simulink model "power_FCHPS_MEA"  (R2020b)
settings: Solver=ode23tb  StartTime=0.0  StopTime=350  RelTol=1e-3  EnableMultiTasking=on
PreLoadFcn:
  | Ts=100e-6;
InitFcn:
  | Ts=100e-6;
undefined symbols (not defined in the file or in its folder): DiscIntNeverNeededParam, Ion, Lithium
libraries: powerlib x93, simulink x8, powerlib_meascontrol x3, electricdrivelib x3
(part 2 of 4)

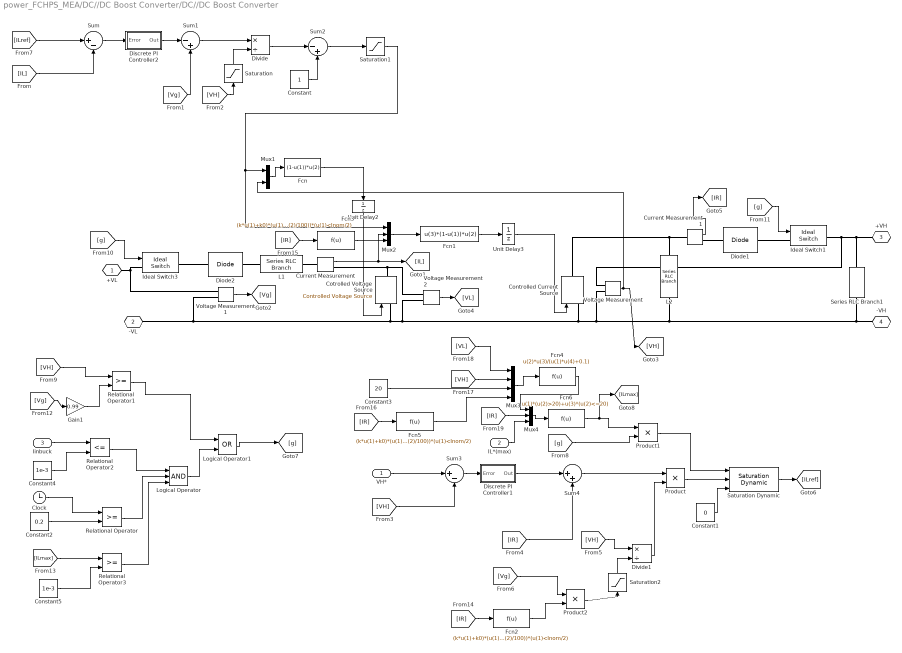
== system power_FCHPS_MEA/DC//DC Boost Converter/DC//DC Boost Converter ==
  VH* : Inport
  IL*(max) : Inport  Port=2
  Iinbuck : Inport  Port=3
  Clock : Clock
  Constant : Constant
  Constant1 : Constant  Value=0
  Constant2 : Constant  Value=0.2
  Constant3 : Constant  Value=20
  Constant4 : Constant  Value=1e-3
  Constant5 : Constant  Value=1e-3
  Controlled Current Source : powerlib/Electrical Sources/Controlled Current Source  Initialize=on  Source_Type=DC  Amplitude=0  Phase=0  Frequency=0  Measurements=None
  Cotrolled Voltage Source : powerlib/Electrical Sources/Controlled Voltage Source  Initialize=on  Source_Type=DC  Amplitude=0  Phase=0  Frequency=0  Measurements=None
  Current Measurement : powerlib/Measurements/Current Measurement  PhasorSimulation=off  OutputType=Complex  PSBequivalent=0
  Current Measurement1 : powerlib/Measurements/Current Measurement  PhasorSimulation=off  OutputType=Complex  PSBequivalent=0
  Diode1 : powerlib/Power Electronics/Diode  Ron=0.001  Lon=0  Vf=0  IC=0  UseSnubber=off  Rs=1e6  Cs=250e-9  Measurements=off
  Diode2 : powerlib/Power Electronics/Diode  Ron=0.001  Lon=0  Vf=0  IC=0  UseSnubber=off  Rs=1e6  Cs=250e-9  Measurements=off
  Discrete PI Controller1 : Subsystem  DialogController=POWERSYS.PowerSysDialog  mask(Discrete PI Controller){Kp=Kpv, Ki=Kiv, Par_Limits=[0.06 -0.06], Init=0, Ts=Ts}
      mask prompts: Kp "Proportional gain (Kp):"; Ki "Integral gain (Ki):"; Par_Limits "Output limits: [ Upper   Lower ]"; Init "Output initial value:"; Ts "Sample time:"
      mask help: This block implements a discrete PI controller.
      mask init:
      | UpperLimit=Par_Limits(1);
      | LowerLimit=Par_Limits(2);
      | power_initmask();
      mask Help: This block is part of a subset of blocks in the Extras library that does not have documentation associated with it, other than the block mask description.
      mask Display: disp('PI');
  Discrete PI Controller2 : Subsystem  DialogController=POWERSYS.PowerSysDialog  mask(Discrete PI Controller){Kp=Kpi, Ki=Kii, Par_Limits=[50 -50], Init=0, Ts=Ts}
      mask prompts: Kp "Proportional gain (Kp):"; Ki "Integral gain (Ki):"; Par_Limits "Output limits: [ Upper   Lower ]"; Init "Output initial value:"; Ts "Sample time:"
      mask help: This block implements a discrete PI controller.
      mask init:
      | UpperLimit=Par_Limits(1);
      | LowerLimit=Par_Limits(2);
      | power_initmask();
      mask Help: This block is part of a subset of blocks in the Extras library that does not have documentation associated with it, other than the block mask description.
      mask Display: disp('PI');
  Divide : Product  Inputs=*/  SampleTime=Ts
  Divide1 : Product  Inputs=*/  SampleTime=Ts
  Fcn : Fcn  Expr=(1-u(1))*u(2)
  Fcn1 : Fcn  Expr=u(3)*(1-u(1))*u(2)
  Fcn2 : Fcn  Expr=(k*u(1)+k0)*(u(1)>=Inom/2)+((n(2)/100))*(u(1)<Inom/2)  SampleTime=Ts
  Fcn3 : Fcn  Expr=(k*u(1)+k0)*(u(1)>=Inom/2)+((n(2)/100))*(u(1)<Inom/2)  SampleTime=Ts
  Fcn4 : Fcn  Expr=u(2)*u(3)/(u(1)*u(4)+0.1)  SampleTime=Ts
  Fcn5 : Fcn  Expr=(k*u(1)+k0)*(u(1)>=Inom/2)+((n(2)/100))*(u(1)<Inom/2)  SampleTime=Ts
  Fcn6 : Fcn  Expr=u(1)*(u(2)>20)+u(3)*(u(2)<=20)  SampleTime=Ts
  Gain1 : Gain  Gain=0.99  SampleTime=Ts
  Ideal Switch1 : powerlib/Power Electronics/Ideal Switch  Ron=0.001  Lon=0  IC=0  Rs=1e5  Cs=inf  Measurements=off
  Ideal Switch3 : powerlib/Power Electronics/Ideal Switch  Ron=0.001  Lon=0  IC=0  Rs=1e5  Cs=inf  Measurements=off
  L1 : powerlib/Elements/Series RLC Branch  LConnTagsString=__new0  RConnTagsString=__new0  BranchType=L  Resistance=0.3  Inductance=L  SetiL0=off  InitialCurrent=100  Capacitance=100e-6  Setx0=off  InitialVoltage=0  Measurements=None
  L2 : powerlib/Elements/Series RLC Branch  LConnTagsString=__new0  RConnTagsString=__new0  BranchType=RC  Resistance=0.01  Inductance=100e-6  SetiL0=off  InitialCurrent=100  Capacitance=800e-6  Setx0=off  InitialVoltage=0  Measurements=None
  Logical Operator : Logic  Inputs=3  AllPortsSameDT=off  OutDataTypeStr=boolean
  Logical Operator1 : Logic  Operator=OR  AllPortsSameDT=off  OutDataTypeStr=boolean
  Mux1 : Mux  Inputs=2
  Mux2 : Mux  Inputs=3
  Mux3 : Mux
  Mux4 : Mux  Inputs=3
  Product : Product  RndMeth=Zero
  Product1 : Product  RndMeth=Zero
  Product2 : Product  RndMeth=Zero
  Relational Operator : RelationalOperator  OutDataTypeStr=boolean  RndMeth=Nearest
  Relational Operator1 : RelationalOperator  OutDataTypeStr=boolean  RndMeth=Nearest
  Relational Operator2 : RelationalOperator  Operator=<=  OutDataTypeStr=boolean  RndMeth=Nearest
  Relational Operator3 : RelationalOperator  OutDataTypeStr=boolean  RndMeth=Nearest
  Saturation : Saturate  UpperLimit=inf  LowerLimit=0.01  SampleTime=Ts
  Saturation Dynamic : simulink/Discontinuities/Saturation Dynamic  OutMin=[]  OutMax=[]  OutDataTypeStr=Inherit: Same as second input  OutDataType=fixdt(1, 16)  OutScaling=2^-10  DoSatur=off
  Saturation1 : Saturate  UpperLimit=1  LowerLimit=0  SampleTime=Ts
  Saturation2 : Saturate  UpperLimit=inf  LowerLimit=0.01  SampleTime=Ts
  Series RLC Branch1 : powerlib/Elements/Series RLC Branch  LConnTagsString=__new0  RConnTagsString=__new0  BranchType=R  Resistance=5e3  Inductance=1e-3  SetiL0=off  InitialCurrent=0  Capacitance=15  Setx0=on  InitialVoltage=270  Measurements=None
  Sum : Sum  Inputs=|+-
  Sum1 : Sum  Inputs=|-+
  Sum2 : Sum  Inputs=|-+
  Sum3 : Sum  Inputs=|+-
  Sum4 : Sum  Inputs=|++
  Unit Delay2 : UnitDelay  SampleTime=Ts  HasFrameUpgradeWarning=on
  Unit Delay3 : UnitDelay  SampleTime=Ts  HasFrameUpgradeWarning=on
  Voltage Measurement : powerlib/Measurements/Voltage Measurement  PhasorSimulation=off  OutputType=Complex  PSBequivalent=0
  Voltage Measurement1 : powerlib/Measurements/Voltage Measurement  PhasorSimulation=off  OutputType=Complex  PSBequivalent=0
  Voltage Measurement2 : powerlib/Measurements/Voltage Measurement  PhasorSimulation=off  OutputType=Complex  PSBequivalent=0
  +VL : PMIOPort  Tag=PMCPort  Side=Left
  -VL : PMIOPort  Tag=PMCPort  Port=2  Side=Left
  +VH : PMIOPort  Tag=PMCPort  Port=3  Side=Right
  -VH : PMIOPort  Tag=PMCPort  Port=4  Side=Right
  wires:
  Voltage Measurement/1 -> [VH], Mux1/2
  Mux1/1 -> Fcn/1
  Fcn/1 -> Unit Delay2/1
  Current Measurement/1 -> Mux2/2, [IL]
  Mux2/1 -> Fcn1/1
  Voltage Measurement1/1 -> [Vg]
  [IL] -> Sum/2
  Sum/1 -> Discrete PI Controller2/1(Error)
  Discrete PI Controller2/1(Out) -> Sum1/1
  [Vg] -> Sum1/2
  Sum1/1 -> Divide/1
  [VH] -> Saturation/1
  Saturation/1 -> Divide/2
  Constant/1 -> Sum2/2
  Sum2/1 -> Saturation1/1
  Saturation1/1 -> Mux1/1, Mux2/1
  [VH] -> Sum3/2
  VH*/1 -> Sum3/1
  Sum3/1 -> Discrete PI Controller1/1(Error)
  Discrete PI Controller1/1(Out) -> Sum4/1
  [IR] -> Sum4/2
  Saturation2/1 -> Divide1/2
  Voltage Measurement2/1 -> [VL]
  Current Measurement1/1 -> [IR]
  Sum4/1 -> Product/1
  [VH] -> Divide1/1
  [Vg] -> Product2/1
  Product2/1 -> Saturation2/1
  Divide1/1 -> Product/2
  Product/1 -> Saturation Dynamic/2
  Constant1/1 -> Saturation Dynamic/3
  Saturation Dynamic/1 -> [ILref]
  Fcn1/1 -> Unit Delay3/1
  [g] -> Ideal Switch3/1
  [g] -> Ideal Switch1/1
  Clock/1 -> Relational Operator/1
  Constant2/1 -> Relational Operator/2
  [g] -> Product1/2
  [VH] -> Relational Operator1/1
  [Vg] -> Gain1/1
  Relational Operator1/1 -> Logical Operator1/1
  Gain1/1 -> Relational Operator1/2
  Product1/1 -> Saturation Dynamic/1
  Iinbuck/1 -> Relational Operator2/1
  Constant4/1 -> Relational Operator2/2
  Relational Operator2/1 -> Logical Operator/1
  Relational Operator/1 -> Logical Operator/2
  Logical Operator/1 -> Logical Operator1/2
  Logical Operator1/1 -> [g]
  [ILmax] -> Relational Operator3/1
  Constant5/1 -> Relational Operator3/2
  Relational Operator3/1 -> Logical Operator/3
  [ILref] -> Sum/1
  Fcn2/1 -> Product2/2
  [IR] -> Fcn3/1
  Fcn3/1 -> Mux2/3
  [IR] -> Fcn2/1
  Constant3/1 -> Mux3/3
  [VH] -> Mux3/2
  [VL] -> Mux3/1
  Mux3/1 -> Fcn4/1
  Fcn5/1 -> Mux3/4
  [IR] -> Fcn5/1
  Fcn4/1 -> Mux4/1
  [IR] -> Mux4/2
  IL*(max)/1 -> Mux4/3
  Mux4/1 -> Fcn6/1
  Fcn6/1 -> Product1/1, [ILmax]
  Unit Delay2/1 -> Cotrolled Voltage Source/1
  Unit Delay3/1 -> Controlled Current Source/1
  Divide/1 -> Sum2/1
  connections:
  Controlled Current Source/RConn1 -- L2/LConn1 -- Current Measurement1/LConn1
  Cotrolled Voltage Source/RConn1 -- Current Measurement/RConn1 -- Voltage Measurement2/LConn1
  L1/LConn1 -- Current Measurement/LConn1
  Diode2/RConn1 -- L1/RConn1
  Current Measurement1/RConn1 -- Diode1/LConn1
  -VH/RConn1 -- Controlled Current Source/LConn1 -- Voltage Measurement2/LConn2 -- Cotrolled Voltage Source/LConn1 -- Voltage Measurement1/LConn2 -- -VL/RConn1 -- Voltage Measurement/LConn2 -- L2/RConn1 -- Series RLC Branch1/RConn1
  Ideal Switch3/RConn1 -- Diode2/LConn1
  +VL/RConn1 -- Voltage Measurement1/LConn1 -- Ideal Switch3/LConn1
  Diode1/RConn1 -- Ideal Switch1/LConn1
  Voltage Measurement/LConn1 -- Ideal Switch1/RConn1 -- +VH/RConn1 -- Series RLC Branch1/LConn1

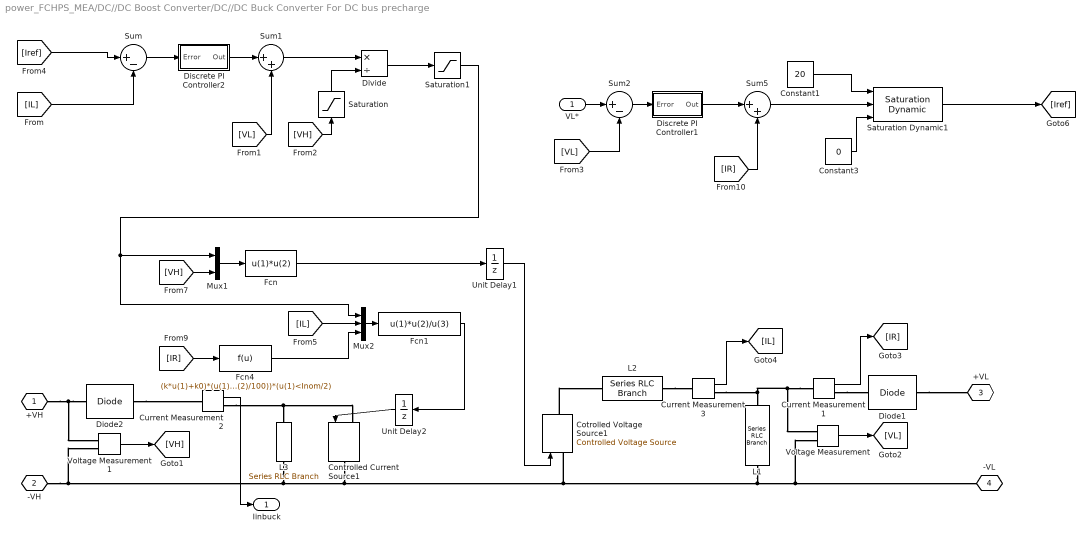
== system power_FCHPS_MEA/DC//DC Boost Converter/DC//DC Buck Converter For DC bus precharge ==
  VL* : Inport
  Constant1 : Constant  Value=20
  Constant3 : Constant  Value=0
  Controlled Current Source1 : powerlib/Electrical Sources/Controlled Current Source  Initialize=on  Source_Type=DC  Amplitude=0  Phase=0  Frequency=0  Measurements=None
  Cotrolled Voltage Source1 : powerlib/Electrical Sources/Controlled Voltage Source  Initialize=on  Source_Type=DC  Amplitude=0  Phase=0  Frequency=0  Measurements=None
  Current Measurement1 : powerlib/Measurements/Current Measurement  PhasorSimulation=off  OutputType=Complex  PSBequivalent=0
  Current Measurement2 : powerlib/Measurements/Current Measurement  PhasorSimulation=off  OutputType=Complex  PSBequivalent=0
  Current Measurement3 : powerlib/Measurements/Current Measurement  PhasorSimulation=off  OutputType=Complex  PSBequivalent=0
  Diode1 : powerlib/Power Electronics/Diode  Ron=0.001  Lon=0  Vf=0  IC=0  UseSnubber=off  Rs=1e6  Cs=250e-9  Measurements=off
  Diode2 : powerlib/Power Electronics/Diode  Ron=0.001  Lon=0  Vf=0  IC=0  UseSnubber=off  Rs=1e6  Cs=250e-9  Measurements=off
  Discrete PI Controller1 : Subsystem  DialogController=POWERSYS.PowerSysDialog  mask(Discrete PI Controller){Kp=Kpv, Ki=Kiv, Par_Limits=[1e6 -1e6], Init=0, Ts=Ts}
      mask prompts: Kp "Proportional gain (Kp):"; Ki "Integral gain (Ki):"; Par_Limits "Output limits: [ Upper   Lower ]"; Init "Output initial value:"; Ts "Sample time:"
      mask help: This block implements a discrete PI controller.
      mask init:
      | UpperLimit=Par_Limits(1);
      | LowerLimit=Par_Limits(2);
      | power_initmask();
      mask Help: This block is part of a subset of blocks in the Extras library that does not have documentation associated with it, other than the block mask description.
      mask Display: disp('PI');
  Discrete PI Controller2 : Subsystem  DialogController=POWERSYS.PowerSysDialog  mask(Discrete PI Controller){Kp=Kpi, Ki=Kii, Par_Limits=[1e6 -1e6], Init=0, Ts=Ts}
      mask prompts: Kp "Proportional gain (Kp):"; Ki "Integral gain (Ki):"; Par_Limits "Output limits: [ Upper   Lower ]"; Init "Output initial value:"; Ts "Sample time:"
      mask help: This block implements a discrete PI controller.
      mask init:
      | UpperLimit=Par_Limits(1);
      | LowerLimit=Par_Limits(2);
      | power_initmask();
      mask Help: This block is part of a subset of blocks in the Extras library that does not have documentation associated with it, other than the block mask description.
      mask Display: disp('PI');
  Divide : Product  Inputs=*/  SampleTime=Ts
  Fcn : Fcn  Expr=u(1)*u(2)
  Fcn1 : Fcn  Expr=u(1)*u(2)/u(3)
  Fcn4 : Fcn  Expr=(k*u(1)+k0)*(u(1)>=Inom/2)+((n(2)/100))*(u(1)<Inom/2)  SampleTime=Ts
  L1 : powerlib/Elements/Series RLC Branch  LConnTagsString=__new0  RConnTagsString=__new0  BranchType=RC  Resistance=0.01  Inductance=10e-6  SetiL0=off  InitialCurrent=100  Capacitance=800e-6  Setx0=off  InitialVoltage=0  Measurements=None
  L2 : powerlib/Elements/Series RLC Branch  LConnTagsString=__new0  RConnTagsString=__new0  BranchType=L  Resistance=0.3  Inductance=L  SetiL0=off  InitialCurrent=100  Capacitance=100e-6  Setx0=off  InitialVoltage=0  Measurements=None
  L3 : powerlib/Elements/Series RLC Branch  LConnTagsString=__new0  RConnTagsString=__new0  BranchType=R  Resistance=1e6  Inductance=10e-6  SetiL0=off  InitialCurrent=100  Capacitance=800e-6  Setx0=off  InitialVoltage=0  Measurements=None
  Mux1 : Mux  Inputs=2
  Mux2 : Mux  Inputs=3
  Saturation : Saturate  UpperLimit=inf  LowerLimit=0.01  SampleTime=Ts
  Saturation Dynamic1 : simulink/Discontinuities/Saturation Dynamic  OutMin=[]  OutMax=[]  OutDataTypeStr=Inherit: Same as second input  OutDataType=fixdt(1, 16)  OutScaling=2^-10  DoSatur=off
  Saturation1 : Saturate  UpperLimit=1  LowerLimit=0  SampleTime=Ts
  Sum : Sum  Inputs=|+-
  Sum1 : Sum  Inputs=|++
  Sum2 : Sum  Inputs=|+-
  Sum5 : Sum  Inputs=|++
  Unit Delay1 : UnitDelay  SampleTime=Ts  HasFrameUpgradeWarning=on
  Unit Delay2 : UnitDelay  SampleTime=Ts  HasFrameUpgradeWarning=on
  Voltage Measurement : powerlib/Measurements/Voltage Measurement  PhasorSimulation=off  OutputType=Complex  PSBequivalent=0
  Voltage Measurement1 : powerlib/Measurements/Voltage Measurement  PhasorSimulation=off  OutputType=Complex  PSBequivalent=0
  +VH : PMIOPort  Tag=PMCPort  Side=Left
  -VH : PMIOPort  Tag=PMCPort  Port=2  Side=Left
  +VL : PMIOPort  Tag=PMCPort  Port=3  Side=Right
  -VL : PMIOPort  Tag=PMCPort  Port=4  Side=Right
  Iinbuck : Outport  VectorParamsAs1DForOutWhenUnconnected=off
  wires:
  Mux2/1 -> Fcn1/1
  Mux1/1 -> Fcn/1
  Voltage Measurement/1 -> [VL]
  Voltage Measurement1/1 -> [VH]
  Current Measurement2/1 -> Iinbuck/1
  Current Measurement1/1 -> [IR]
  [IL] -> Mux2/2
  [VH] -> Mux1/2
  Fcn/1 -> Unit Delay1/1
  Fcn1/1 -> Unit Delay2/1
  [IL] -> Sum/2
  Sum/1 -> Discrete PI Controller2/1(Error)
  Discrete PI Controller2/1(Out) -> Sum1/1
  [VL] -> Sum1/2
  Sum1/1 -> Divide/1
  [VH] -> Saturation/1
  Saturation/1 -> Divide/2
  Divide/1 -> Saturation1/1
  Saturation1/1 -> Mux2/1, Mux1/1
  [Iref] -> Sum/1
  Sum2/1 -> Discrete PI Controller1/1(Error)
  Discrete PI Controller1/1(Out) -> Sum5/1
  [IR] -> Sum5/2
  Sum5/1 -> Saturation Dynamic1/2
  Constant3/1 -> Saturation Dynamic1/3
  Saturation Dynamic1/1 -> [Iref]
  VL*/1 -> Sum2/1
  [VL] -> Sum2/2
  Current Measurement3/1 -> [IL]
  [IR] -> Fcn4/1
  Fcn4/1 -> Mux2/3
  Constant1/1 -> Saturation Dynamic1/1
  Unit Delay1/1 -> Cotrolled Voltage Source1/1
  Unit Delay2/1 -> Controlled Current Source1/1
  connections:
  -VH/RConn1 -- Voltage Measurement1/LConn2 -- Cotrolled Voltage Source1/LConn1 -- L1/RConn1 -- -VL/RConn1 -- Voltage Measurement/LConn2 -- Controlled Current Source1/RConn1 -- L3/RConn1
  Diode2/LConn1 -- +VH/RConn1 -- Voltage Measurement1/LConn1
  Cotrolled Voltage Source1/RConn1 -- L2/RConn1
  Current Measurement1/LConn1 -- Voltage Measurement/LConn1 -- Current Measurement3/RConn1 -- L1/LConn1
  Current Measurement1/RConn1 -- Diode1/LConn1
  Diode1/RConn1 -- +VL/RConn1
  Current Measurement2/RConn1 -- Controlled Current Source1/LConn1 -- L3/LConn1
  L2/LConn1 -- Current Measurement3/LConn1
  Diode2/RConn1 -- Current Measurement2/LConn1

== system power_FCHPS_MEA/DC//DC Buck Converter/Discrete PI Controller1 ==
  note: Discrete PID Controller
  note: Pierre Giroux, Gilbert Sybille
      | Power System Simulation Laboratory
      | IREQ, Hydro-Quebc
  Error : Inport  SampleTime=Ts
  Discrete-Time Integrator : DiscreteIntegrator  InitialCondition=Init  SampleTime=Ts  LimitOutput=on  UpperSaturationLimit=UpperLimit  LowerSaturationLimit=LowerLimit  ICPrevOutput=DiscIntNeverNeededParam  ICPrevScaledInput=DiscIntNeverNeededParam
  Kp4 : Gain  Gain=Kp  SaturateOnIntegerOverflow=on  SampleTime=Ts  OutDataTypeStr=Inherit: Same as input  ParamDataTypeStr=Inherit: Same as input
  Kp5 : Gain  Gain=Ki  SaturateOnIntegerOverflow=on  SampleTime=Ts  OutDataTypeStr=Inherit: Same as input  ParamDataTypeStr=Inherit: Same as input
  Saturation2 : Saturate  UpperLimit=UpperLimit  LowerLimit=LowerLimit  SampleTime=Ts
  Sum6 : Sum  InputSameDT=on  SaturateOnIntegerOverflow=on  SampleTime=Ts  OutDataTypeStr=Inherit: Same as first input
  Zero-Order Hold : ZeroOrderHold  SampleTime=Ts
  Out : Outport  SampleTime=Ts  InitialOutput=0  VectorParamsAs1DForOutWhenUnconnected=off
  wires:
  Zero-Order Hold/1 -> Sum6/1
  Saturation2/1 -> Out/1
  Discrete-Time Integrator/1 -> Sum6/2
  Kp4/1 -> Zero-Order Hold/1
  Kp5/1 -> Discrete-Time Integrator/1
  Sum6/1 -> Saturation2/1
  Error/1 -> Kp5/1, Kp4/1

== system power_FCHPS_MEA/DC//DC Buck Converter/Discrete PI Controller2 ==
  note: Pierre Giroux, Gilbert Sybille
      | Power System Simulation Laboratory
      | IREQ, Hydro-Quebc
  note: Discrete PID Controller
  Error : Inport  SampleTime=Ts
  Discrete-Time Integrator : DiscreteIntegrator  InitialCondition=Init  SampleTime=Ts  LimitOutput=on  UpperSaturationLimit=UpperLimit  LowerSaturationLimit=LowerLimit  ICPrevOutput=DiscIntNeverNeededParam  ICPrevScaledInput=DiscIntNeverNeededParam
  Kp4 : Gain  Gain=Kp  SaturateOnIntegerOverflow=on  SampleTime=Ts  OutDataTypeStr=Inherit: Same as input  ParamDataTypeStr=Inherit: Same as input
  Kp5 : Gain  Gain=Ki  SaturateOnIntegerOverflow=on  SampleTime=Ts  OutDataTypeStr=Inherit: Same as input  ParamDataTypeStr=Inherit: Same as input
  Saturation2 : Saturate  UpperLimit=UpperLimit  LowerLimit=LowerLimit  SampleTime=Ts
  Sum6 : Sum  InputSameDT=on  SaturateOnIntegerOverflow=on  SampleTime=Ts  OutDataTypeStr=Inherit: Same as first input
  Zero-Order Hold : ZeroOrderHold  SampleTime=Ts
  Out : Outport  SampleTime=Ts  InitialOutput=0  VectorParamsAs1DForOutWhenUnconnected=off
  wires:
  Error/1 -> Kp4/1, Kp5/1
  Sum6/1 -> Saturation2/1
  Kp5/1 -> Discrete-Time Integrator/1
  Kp4/1 -> Zero-Order Hold/1
  Discrete-Time Integrator/1 -> Sum6/2
  Saturation2/1 -> Out/1
  Zero-Order Hold/1 -> Sum6/1

== system power_FCHPS_MEA/Energy Management System/Battery DC//DC charge converter reference ==
  IBAT* : Inport
  Constant1 : Constant  Value=0
  Constant8 : Constant  Value=58
  Switch5 : Switch  Criteria=u2 > Threshold
  IBAT_maxC* : Outport  VectorParamsAs1DForOutWhenUnconnected=off
  VBAT* : Outport  Port=2  VectorParamsAs1DForOutWhenUnconnected=off
  wires:
  [EMSON] -> Switch5/2
  IBAT*/1 -> Switch5/1
  Constant1/1 -> Switch5/3
  Switch5/1 -> IBAT_maxC*/1
  Constant8/1 -> VBAT*/1

== system power_FCHPS_MEA/Energy Management System/Battery DC//DC discharge converter references  ==
  IBAT* : Inport
  Constant10 : Constant  Value=0
  Constant6 : Constant  Value=270
  Switch1 : Switch  Criteria=u2 > Threshold
  Switch10 : Switch  Criteria=u2 > Threshold
  IBAT_maxD* : Outport  VectorParamsAs1DForOutWhenUnconnected=off
  VDC2* : Outport  Port=2  VectorParamsAs1DForOutWhenUnconnected=off
  wires:
  Switch10/1 -> VDC2*/1
  [EMSON] -> Switch10/2
  Constant6/1 -> Switch10/3
  IBAT*/1 -> Switch1/1
  [Vdcref] -> Switch10/1
  [EMSON] -> Switch1/2
  Switch1/1 -> IBAT_maxD*/1
  Constant10/1 -> Switch1/3

== system power_FCHPS_MEA/Energy Management System/FC DC//DC converter references ==
  IFC* : Inport
  Add1 : Sum  Inputs=+-
  Constant11 : Constant  Value=212
  Constant22 : Constant  Value=270
  Constant3 : Constant  Value=15
  Constant4 : Constant  Value=297
  Constant7 : Constant  Value=250
  Fcn : Fcn  Expr=u(1)*(u(1)<u(2))+u(2)*(u(1)>=u(2))
  Mux6 : Mux  Inputs=2
  Relational Operator6 : RelationalOperator  Operator=<=  OutDataTypeStr=boolean  RndMeth=Nearest
  Switch : Switch  Criteria=u2 > Threshold
  Switch6 : Switch  Criteria=u2 > Threshold
  Switch9 : Switch  Criteria=u2 > Threshold
  filter : Subsystem
  IFC*max : Outport  VectorParamsAs1DForOutWhenUnconnected=off
  VDC1* : Outport  Port=2  VectorParamsAs1DForOutWhenUnconnected=off
  wires:
  [EMSON] -> Switch9/2
  Switch9/1 -> VDC1*/1
  Constant4/1 -> Switch9/1
  Constant22/1 -> Switch9/3
  Switch6/1 -> Switch/1
  Constant11/1 -> Relational Operator6/2, Switch6/3
  Relational Operator6/1 -> Switch6/2
  Constant7/1 -> Switch/3
  Constant3/1 -> Add1/2
  IFC*/1 -> Relational Operator6/1, Switch6/1
  Mux6/1 -> Fcn/1
  Fcn/1 -> filter/1(I)
  [EMSON] -> Switch/2
  Switch/1 -> Mux6/1
  filter/1(If) -> IFC*max/1
  Add1/1 -> Mux6/2
  [IFCAllow] -> Add1/1

== system power_FCHPS_MEA/Energy Management System/Load Disconnect ==
  SOC : Inport
  Vdc : Inport  Port=2
  Constant17 : Constant  Value=40
  Constant18 : Constant  Value=0
  Constant19 : Constant  Value=0
  Constant2 : Constant  Value=270
  Constant5 : Constant
  Constant9 : Constant  Value=200
  Data Type Conversion2 : DataTypeConversion
  Logical Operator3 : Logic  AllPortsSameDT=off  OutDataTypeStr=boolean
  Relational Operator : RelationalOperator  OutDataTypeStr=boolean  RndMeth=Nearest
  Relational Operator3 : RelationalOperator  Operator=<=  OutDataTypeStr=boolean  RndMeth=Nearest
  Relational Operator5 : RelationalOperator  Operator=<=  OutDataTypeStr=boolean  RndMeth=Nearest
  Switch2 : Switch  Criteria=u2 > Threshold
  Switch7 : Switch  Criteria=u2 > Threshold
  Switch8 : Switch  Criteria=u2 > Threshold
  Unit Delay : UnitDelay  SampleTime=Ts  HasFrameUpgradeWarning=on
  Unit Delay4 : UnitDelay  InitialCondition=1  SampleTime=Ts  HasFrameUpgradeWarning=on
  LoadON : Outport  VectorParamsAs1DForOutWhenUnconnected=off
  tag scope: EMSON=global
  wires:
  Data Type Conversion2/1 -> LoadON/1
  Relational Operator3/1 -> Switch8/2
  Constant18/1 -> Switch7/1
  Switch8/1 -> Switch2/3
  Relational Operator5/1 -> Switch7/2
  Constant17/1 -> Relational Operator5/2
  Switch7/1 -> Unit Delay4/1, Logical Operator3/1
  Unit Delay4/1 -> Switch7/3
  Unit Delay/1 -> Switch8/3
  SOC/1 -> Relational Operator5/1
  Logical Operator3/1 -> Data Type Conversion2/1
  Constant19/1 -> Switch8/1
  Constant9/1 -> Relational Operator3/2
  Relational Operator/1 -> Switch2/2
  Constant5/1 -> Switch2/1
  Constant2/1 -> Relational Operator/2
  Switch2/1 -> [EMSON], Unit Delay/1, Logical Operator3/2
  Vdc/1 -> Relational Operator/1, Relational Operator3/1

== system power_FCHPS_MEA/Energy Management System/Model ==
  Pload : Inport
  SOC : Inport  Port=2
  Classical PI Control : Subsystem  VariantControl=ClassicalPI
  ECMS Control : Subsystem  VariantControl=ECMS
  EEMS Control : Subsystem  VariantControl=EEMS
  Frequency Decoupling and State Machine Control : Subsystem  VariantControl=FrequencyDecoupling
  State Machine Control : Subsystem  VariantControl=RuleBasedFuzzyLogic
  IFC* : Outport  VectorParamsAs1DForOutWhenUnconnected=off
  IBATD* : Outport  Port=2  VectorParamsAs1DForOutWhenUnconnected=off
  IBATC* : Outport  Port=3  VectorParamsAs1DForOutWhenUnconnected=off

== system power_FCHPS_MEA/Energy Management System/Protecting resistor connect ==
  Vdc : Inport
  Constant12 : Constant  Value=290
  Constant13 : Constant
  Constant14 : Constant  Value=285
  Constant15 : Constant  Value=0
  Data Type Conversion1 : DataTypeConversion
  Relational Operator1 : RelationalOperator  OutDataTypeStr=boolean  RndMeth=Nearest
  Relational Operator2 : RelationalOperator  Operator=<=  OutDataTypeStr=boolean  RndMeth=Nearest
  Switch3 : Switch  Criteria=u2 > Threshold
  Switch4 : Switch  Criteria=u2 > Threshold
  Unit Delay1 : UnitDelay  SampleTime=Ts  HasFrameUpgradeWarning=on
  ResON : Outport  VectorParamsAs1DForOutWhenUnconnected=off
  wires:
  Unit Delay1/1 -> Switch4/3
  Vdc/1 -> Relational Operator1/1, Relational Operator2/1
  Switch4/1 -> Switch3/3
  Switch3/1 -> Data Type Conversion1/1, Unit Delay1/1
  Relational Operator1/1 -> Switch3/2
  Relational Operator2/1 -> Switch4/2
  Data Type Conversion1/1 -> ResON/1
  Constant15/1 -> Switch4/1
  Constant13/1 -> Switch3/1
  Constant14/1 -> Relational Operator2/2
  Constant12/1 -> Relational Operator1/2

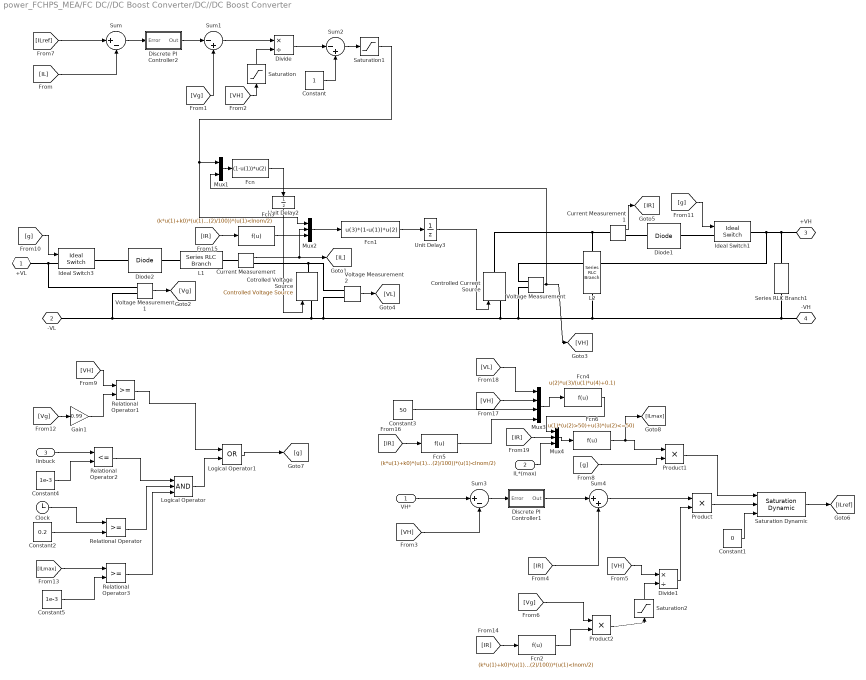
== system power_FCHPS_MEA/FC DC//DC Boost Converter/DC//DC Boost Converter ==
  VH* : Inport
  IL*(max) : Inport  Port=2
  Iinbuck : Inport  Port=3
  Clock : Clock
  Constant : Constant
  Constant1 : Constant  Value=0
  Constant2 : Constant  Value=0.2
  Constant3 : Constant  Value=50
  Constant4 : Constant  Value=1e-3
  Constant5 : Constant  Value=1e-3
  Controlled Current Source : powerlib/Electrical Sources/Controlled Current Source  Initialize=on  Source_Type=DC  Amplitude=0  Phase=0  Frequency=0  Measurements=None
  Cotrolled Voltage Source : powerlib/Electrical Sources/Controlled Voltage Source  Initialize=on  Source_Type=DC  Amplitude=0  Phase=0  Frequency=0  Measurements=None
  Current Measurement : powerlib/Measurements/Current Measurement  PhasorSimulation=off  OutputType=Complex  PSBequivalent=0
  Current Measurement1 : powerlib/Measurements/Current Measurement  PhasorSimulation=off  OutputType=Complex  PSBequivalent=0
  Diode1 : powerlib/Power Electronics/Diode  Ron=0.001  Lon=0  Vf=0  IC=0  UseSnubber=off  Rs=1e6  Cs=250e-9  Measurements=off
  Diode2 : powerlib/Power Electronics/Diode  Ron=0.001  Lon=0  Vf=0  IC=0  UseSnubber=off  Rs=1e6  Cs=250e-9  Measurements=off
  Discrete PI Controller1 : Subsystem  DialogController=POWERSYS.PowerSysDialog  mask(Discrete PI Controller){Kp=Kpv, Ki=Kiv, Par_Limits=[0.5 -0.5], Init=0, Ts=Ts}
      mask prompts: Kp "Proportional gain (Kp):"; Ki "Integral gain (Ki):"; Par_Limits "Output limits: [ Upper   Lower ]"; Init "Output initial value:"; Ts "Sample time:"
      mask help: This block implements a discrete PI controller.
      mask init:
      | UpperLimit=Par_Limits(1);
      | LowerLimit=Par_Limits(2);
      | power_initmask();
      mask Help: This block is part of a subset of blocks in the Extras library that does not have documentation associated with it, other than the block mask description.
      mask Display: disp('PI');
  Discrete PI Controller2 : Subsystem  DialogController=POWERSYS.PowerSysDialog  mask(Discrete PI Controller){Kp=Kpi/1000, Ki=Kii/1000, Par_Limits=[50 -50], Init=0, Ts=Ts}
      mask prompts: Kp "Proportional gain (Kp):"; Ki "Integral gain (Ki):"; Par_Limits "Output limits: [ Upper   Lower ]"; Init "Output initial value:"; Ts "Sample time:"
      mask help: This block implements a discrete PI controller.
      mask init:
      | UpperLimit=Par_Limits(1);
      | LowerLimit=Par_Limits(2);
      | power_initmask();
      mask Help: This block is part of a subset of blocks in the Extras library that does not have documentation associated with it, other than the block mask description.
      mask Display: disp('PI');
  Divide : Product  Inputs=*/  SampleTime=Ts
  Divide1 : Product  Inputs=*/  SampleTime=Ts
  Fcn : Fcn  Expr=(1-u(1))*u(2)
  Fcn1 : Fcn  Expr=u(3)*(1-u(1))*u(2)
  Fcn2 : Fcn  Expr=(k*u(1)+k0)*(u(1)>=Inom/2)+((n(2)/100))*(u(1)<Inom/2)  SampleTime=Ts
  Fcn3 : Fcn  Expr=(k*u(1)+k0)*(u(1)>=Inom/2)+((n(2)/100))*(u(1)<Inom/2)  SampleTime=Ts
  Fcn4 : Fcn  Expr=u(2)*u(3)/(u(1)*u(4)+0.1)  SampleTime=Ts
  Fcn5 : Fcn  Expr=(k*u(1)+k0)*(u(1)>=Inom/2)+((n(2)/100))*(u(1)<Inom/2)  SampleTime=Ts
  Fcn6 : Fcn  Expr=u(1)*(u(2)>50)+u(3)*(u(2)<=50)  SampleTime=Ts
  Gain1 : Gain  Gain=0.99  SampleTime=Ts
  Ideal Switch1 : powerlib/Power Electronics/Ideal Switch  Ron=0.001  Lon=0  IC=0  Rs=1e5  Cs=inf  Measurements=off
  Ideal Switch3 : powerlib/Power Electronics/Ideal Switch  Ron=0.001  Lon=0  IC=0  Rs=1e5  Cs=inf  Measurements=off
  L1 : powerlib/Elements/Series RLC Branch  LConnTagsString=__new0  RConnTagsString=__new0  BranchType=L  Resistance=0.3  Inductance=L  SetiL0=off  InitialCurrent=100  Capacitance=100e-6  Setx0=off  InitialVoltage=0  Measurements=None
  L2 : powerlib/Elements/Series RLC Branch  LConnTagsString=__new0  RConnTagsString=__new0  BranchType=RC  Resistance=0.01  Inductance=100e-6  SetiL0=off  InitialCurrent=100  Capacitance=800e-6  Setx0=off  InitialVoltage=0  Measurements=None
  Logical Operator : Logic  Inputs=3  AllPortsSameDT=off  OutDataTypeStr=boolean
  Logical Operator1 : Logic  Operator=OR  AllPortsSameDT=off  OutDataTypeStr=boolean
  Mux1 : Mux  Inputs=2
  Mux2 : Mux  Inputs=3
  Mux3 : Mux
  Mux4 : Mux  Inputs=3
  Product : Product  RndMeth=Zero
  Product1 : Product  RndMeth=Zero
  Product2 : Product  RndMeth=Zero
  Relational Operator : RelationalOperator  OutDataTypeStr=boolean  RndMeth=Nearest
  Relational Operator1 : RelationalOperator  OutDataTypeStr=boolean  RndMeth=Nearest
  Relational Operator2 : RelationalOperator  Operator=<=  OutDataTypeStr=boolean  RndMeth=Nearest
  Relational Operator3 : RelationalOperator  OutDataTypeStr=boolean  RndMeth=Nearest
  Saturation : Saturate  UpperLimit=inf  LowerLimit=0.01  SampleTime=Ts
  Saturation Dynamic : simulink/Discontinuities/Saturation Dynamic  OutMin=[]  OutMax=[]  OutDataTypeStr=Inherit: Same as second input  OutDataType=fixdt(1, 16)  OutScaling=2^-10  DoSatur=off
  Saturation1 : Saturate  UpperLimit=1  LowerLimit=0  SampleTime=Ts
  Saturation2 : Saturate  UpperLimit=inf  LowerLimit=0.01  SampleTime=Ts
  Series RLC Branch1 : powerlib/Elements/Series RLC Branch  LConnTagsString=__new0  RConnTagsString=__new0  BranchType=R  Resistance=5e3  Inductance=1e-3  SetiL0=off  InitialCurrent=0  Capacitance=15  Setx0=on  InitialVoltage=270  Measurements=None
  Sum : Sum  Inputs=|+-
  Sum1 : Sum  Inputs=|-+
  Sum2 : Sum  Inputs=|-+
  Sum3 : Sum  Inputs=|+-
  Sum4 : Sum  Inputs=|++
  Unit Delay2 : UnitDelay  SampleTime=Ts  HasFrameUpgradeWarning=on
  Unit Delay3 : UnitDelay  SampleTime=Ts  HasFrameUpgradeWarning=on
  Voltage Measurement : powerlib/Measurements/Voltage Measurement  PhasorSimulation=off  OutputType=Complex  PSBequivalent=0
  Voltage Measurement1 : powerlib/Measurements/Voltage Measurement  PhasorSimulation=off  OutputType=Complex  PSBequivalent=0
  Voltage Measurement2 : powerlib/Measurements/Voltage Measurement  PhasorSimulation=off  OutputType=Complex  PSBequivalent=0
  +VL : PMIOPort  Tag=PMCPort  Side=Left
  -VL : PMIOPort  Tag=PMCPort  Port=2  Side=Left
  +VH : PMIOPort  Tag=PMCPort  Port=3  Side=Right
  -VH : PMIOPort  Tag=PMCPort  Port=4  Side=Right
  wires:
  Unit Delay3/1 -> Controlled Current Source/1
  Unit Delay2/1 -> Cotrolled Voltage Source/1
  Fcn6/1 -> [ILmax], Product1/1
  Mux4/1 -> Fcn6/1
  IL*(max)/1 -> Mux4/3
  [IR] -> Mux4/2
  Fcn4/1 -> Mux4/1
  [IR] -> Fcn5/1
  Fcn5/1 -> Mux3/4
  Mux3/1 -> Fcn4/1
  [VL] -> Mux3/1
  [VH] -> Mux3/2
  Constant3/1 -> Mux3/3
  [IR] -> Fcn2/1
  Fcn3/1 -> Mux2/3
  Fcn2/1 -> Product2/2
  [ILref] -> Sum/1
  Relational Operator3/1 -> Logical Operator/3
  Constant5/1 -> Relational Operator3/2
  [ILmax] -> Relational Operator3/1
  Logical Operator1/1 -> [g]
  Logical Operator/1 -> Logical Operator1/2
  Relational Operator/1 -> Logical Operator/2
  Relational Operator2/1 -> Logical Operator/1
  Constant4/1 -> Relational Operator2/2
  Iinbuck/1 -> Relational Operator2/1
  Product1/1 -> Saturation Dynamic/1
  Gain1/1 -> Relational Operator1/2
  Relational Operator1/1 -> Logical Operator1/1
  [Vg] -> Gain1/1
  [VH] -> Relational Operator1/1
  [g] -> Product1/2
  Constant2/1 -> Relational Operator/2
  Clock/1 -> Relational Operator/1
  [g] -> Ideal Switch1/1
  [g] -> Ideal Switch3/1
  Fcn1/1 -> Unit Delay3/1
  Saturation Dynamic/1 -> [ILref]
  Constant1/1 -> Saturation Dynamic/3
  Product/1 -> Saturation Dynamic/2
  Divide1/1 -> Product/2
  Product2/1 -> Saturation2/1
  [Vg] -> Product2/1
  [VH] -> Divide1/1
  Sum4/1 -> Product/1
  Current Measurement1/1 -> [IR]
  Voltage Measurement2/1 -> [VL]
  Saturation2/1 -> Divide1/2
  [IR] -> Sum4/2
  Discrete PI Controller1/1(Out) -> Sum4/1
  Sum3/1 -> Discrete PI Controller1/1(Error)
  VH*/1 -> Sum3/1
  [VH] -> Sum3/2
  Sum2/1 -> Saturation1/1
  Constant/1 -> Sum2/2
  Saturation/1 -> Divide/2
  [VH] -> Saturation/1
  Sum1/1 -> Divide/1
  [Vg] -> Sum1/2
  Discrete PI Controller2/1(Out) -> Sum1/1
  Sum/1 -> Discrete PI Controller2/1(Error)
  [IL] -> Sum/2
  Voltage Measurement1/1 -> [Vg]
  Mux2/1 -> Fcn1/1
  Current Measurement/1 -> [IL], Mux2/2
  Fcn/1 -> Unit Delay2/1
  Mux1/1 -> Fcn/1
  Voltage Measurement/1 -> [VH], Mux1/2
  [IR] -> Fcn3/1
  Divide/1 -> Sum2/1
  Saturation1/1 -> Mux2/1, Mux1/1
  connections:
  Series RLC Branch1/LConn1 -- +VH/RConn1 -- Ideal Switch1/RConn1 -- Voltage Measurement/LConn1
  Diode1/RConn1 -- Ideal Switch1/LConn1
  +VL/RConn1 -- Voltage Measurement1/LConn1 -- Ideal Switch3/LConn1
  Ideal Switch3/RConn1 -- Diode2/LConn1
  Series RLC Branch1/RConn1 -- L2/RConn1 -- Voltage Measurement/LConn2 -- -VL/RConn1 -- Voltage Measurement1/LConn2 -- Cotrolled Voltage Source/LConn1 -- Voltage Measurement2/LConn2 -- Controlled Current Source/LConn1 -- -VH/RConn1
  Current Measurement1/RConn1 -- Diode1/LConn1
  Diode2/RConn1 -- L1/RConn1
  L1/LConn1 -- Current Measurement/LConn1
  Current Measurement/RConn1 -- Voltage Measurement2/LConn1 -- Cotrolled Voltage Source/RConn1
  Current Measurement1/LConn1 -- L2/LConn1 -- Controlled Current Source/RConn1

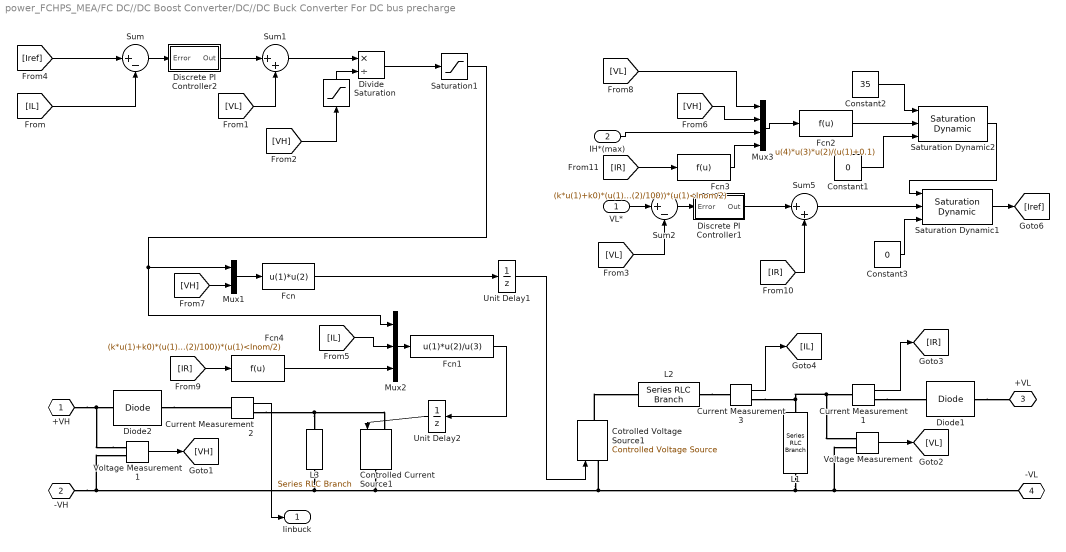
== system power_FCHPS_MEA/FC DC//DC Boost Converter/DC//DC Buck Converter For DC bus precharge ==
  VL* : Inport
  IH*(max) : Inport  Port=2
  Constant1 : Constant  Value=0
  Constant2 : Constant  Value=35
  Constant3 : Constant  Value=0
  Controlled Current Source1 : powerlib/Electrical Sources/Controlled Current Source  Initialize=on  Source_Type=DC  Amplitude=0  Phase=0  Frequency=0  Measurements=None
  Cotrolled Voltage Source1 : powerlib/Electrical Sources/Controlled Voltage Source  Initialize=on  Source_Type=DC  Amplitude=0  Phase=0  Frequency=0  Measurements=None
  Current Measurement1 : powerlib/Measurements/Current Measurement  PhasorSimulation=off  OutputType=Complex  PSBequivalent=0
  Current Measurement2 : powerlib/Measurements/Current Measurement  PhasorSimulation=off  OutputType=Complex  PSBequivalent=0
  Current Measurement3 : powerlib/Measurements/Current Measurement  PhasorSimulation=off  OutputType=Complex  PSBequivalent=0
  Diode1 : powerlib/Power Electronics/Diode  Ron=0.001  Lon=0  Vf=0  IC=0  UseSnubber=off  Rs=1e6  Cs=250e-9  Measurements=off
  Diode2 : powerlib/Power Electronics/Diode  Ron=0.001  Lon=0  Vf=0  IC=0  UseSnubber=off  Rs=1e6  Cs=250e-9  Measurements=off
  Discrete PI Controller1 : Subsystem  DialogController=POWERSYS.PowerSysDialog  mask(Discrete PI Controller){Kp=Kpv, Ki=Kiv, Par_Limits=[1e6 -1e6], Init=0, Ts=Ts}
      mask prompts: Kp "Proportional gain (Kp):"; Ki "Integral gain (Ki):"; Par_Limits "Output limits: [ Upper   Lower ]"; Init "Output initial value:"; Ts "Sample time:"
      mask help: This block implements a discrete PI controller.
      mask init:
      | UpperLimit=Par_Limits(1);
      | LowerLimit=Par_Limits(2);
      | power_initmask();
      mask Help: This block is part of a subset of blocks in the Extras library that does not have documentation associated with it, other than the block mask description.
      mask Display: disp('PI');
  Discrete PI Controller2 : Subsystem  DialogController=POWERSYS.PowerSysDialog  mask(Discrete PI Controller){Kp=Kpi, Ki=Kii, Par_Limits=[1e6 -1e6], Init=0, Ts=Ts}
      mask prompts: Kp "Proportional gain (Kp):"; Ki "Integral gain (Ki):"; Par_Limits "Output limits: [ Upper   Lower ]"; Init "Output initial value:"; Ts "Sample time:"
      mask help: This block implements a discrete PI controller.
      mask init:
      | UpperLimit=Par_Limits(1);
      | LowerLimit=Par_Limits(2);
      | power_initmask();
      mask Help: This block is part of a subset of blocks in the Extras library that does not have documentation associated with it, other than the block mask description.
      mask Display: disp('PI');
  Divide : Product  Inputs=*/  SampleTime=Ts
  Fcn : Fcn  Expr=u(1)*u(2)
  Fcn1 : Fcn  Expr=u(1)*u(2)/u(3)
  Fcn2 : Fcn  Expr=u(4)*u(3)*u(2)/(u(1)+0.1)  SampleTime=Ts
  Fcn3 : Fcn  Expr=(k*u(1)+k0)*(u(1)>=Inom/2)+((n(2)/100))*(u(1)<Inom/2)  SampleTime=Ts
  Fcn4 : Fcn  Expr=(k*u(1)+k0)*(u(1)>=Inom/2)+((n(2)/100))*(u(1)<Inom/2)  SampleTime=Ts
  L1 : powerlib/Elements/Series RLC Branch  LConnTagsString=__new0  RConnTagsString=__new0  BranchType=RC  Resistance=0.01  Inductance=10e-6  SetiL0=off  InitialCurrent=100  Capacitance=800e-6  Setx0=off  InitialVoltage=0  Measurements=None
  L2 : powerlib/Elements/Series RLC Branch  LConnTagsString=__new0  RConnTagsString=__new0  BranchType=L  Resistance=0.3  Inductance=L  SetiL0=off  InitialCurrent=100  Capacitance=100e-6  Setx0=off  InitialVoltage=0  Measurements=None
  L3 : powerlib/Elements/Series RLC Branch  LConnTagsString=__new0  RConnTagsString=__new0  BranchType=R  Resistance=1e6  Inductance=10e-6  SetiL0=off  InitialCurrent=100  Capacitance=800e-6  Setx0=off  InitialVoltage=0  Measurements=None
  Mux1 : Mux  Inputs=2
  Mux2 : Mux  Inputs=3
  Mux3 : Mux
  Saturation : Saturate  UpperLimit=inf  LowerLimit=0.01  SampleTime=Ts
  Saturation Dynamic1 : simulink/Discontinuities/Saturation Dynamic  OutMin=[]  OutMax=[]  OutDataTypeStr=Inherit: Same as second input  OutDataType=fixdt(1, 16)  OutScaling=2^-10  DoSatur=off
  Saturation Dynamic2 : simulink/Discontinuities/Saturation Dynamic  OutMin=[]  OutMax=[]  OutDataTypeStr=Inherit: Same as second input  OutDataType=fixdt(1, 16)  OutScaling=2^-10  DoSatur=off
  Saturation1 : Saturate  UpperLimit=1  LowerLimit=0  SampleTime=Ts
  Sum : Sum  Inputs=|+-
  Sum1 : Sum  Inputs=|++
  Sum2 : Sum  Inputs=|+-
  Sum5 : Sum  Inputs=|++
  Unit Delay1 : UnitDelay  SampleTime=Ts  HasFrameUpgradeWarning=on
  Unit Delay2 : UnitDelay  SampleTime=Ts  HasFrameUpgradeWarning=on
  Voltage Measurement : powerlib/Measurements/Voltage Measurement  PhasorSimulation=off  OutputType=Complex  PSBequivalent=0
  Voltage Measurement1 : powerlib/Measurements/Voltage Measurement  PhasorSimulation=off  OutputType=Complex  PSBequivalent=0
  +VH : PMIOPort  Tag=PMCPort  Side=Left
  -VH : PMIOPort  Tag=PMCPort  Port=2  Side=Left
  +VL : PMIOPort  Tag=PMCPort  Port=3  Side=Right
  -VL : PMIOPort  Tag=PMCPort  Port=4  Side=Right
  Iinbuck : Outport  VectorParamsAs1DForOutWhenUnconnected=off
  wires:
  Unit Delay2/1 -> Controlled Current Source1/1
  Unit Delay1/1 -> Cotrolled Voltage Source1/1
  Fcn4/1 -> Mux2/3
  [IR] -> Fcn4/1
  Current Measurement3/1 -> [IL]
  [VL] -> Sum2/2
  VL*/1 -> Sum2/1
  Saturation Dynamic1/1 -> [Iref]
  Constant3/1 -> Saturation Dynamic1/3
  Sum5/1 -> Saturation Dynamic1/2
  [IR] -> Sum5/2
  Discrete PI Controller1/1(Out) -> Sum5/1
  Sum2/1 -> Discrete PI Controller1/1(Error)
  [Iref] -> Sum/1
  Saturation1/1 -> Mux1/1, Mux2/1
  Divide/1 -> Saturation1/1
  Saturation/1 -> Divide/2
  [VH] -> Saturation/1
  Sum1/1 -> Divide/1
  [VL] -> Sum1/2
  Discrete PI Controller2/1(Out) -> Sum1/1
  Sum/1 -> Discrete PI Controller2/1(Error)
  [IL] -> Sum/2
  Fcn1/1 -> Unit Delay2/1
  Fcn/1 -> Unit Delay1/1
  [VH] -> Mux1/2
  [IL] -> Mux2/2
  Current Measurement1/1 -> [IR]
  Current Measurement2/1 -> Iinbuck/1
  Voltage Measurement1/1 -> [VH]
  Voltage Measurement/1 -> [VL]
  Mux1/1 -> Fcn/1
  Mux2/1 -> Fcn1/1
  IH*(max)/1 -> Mux3/3
  [VH] -> Mux3/2
  [VL] -> Mux3/1
  Mux3/1 -> Fcn2/1
  [IR] -> Fcn3/1
  Fcn3/1 -> Mux3/4
  Fcn2/1 -> Saturation Dynamic2/2
  Saturation Dynamic2/1 -> Saturation Dynamic1/1
  Constant1/1 -> Saturation Dynamic2/3
  Constant2/1 -> Saturation Dynamic2/1
  connections:
  Diode2/RConn1 -- Current Measurement2/LConn1
  L2/LConn1 -- Current Measurement3/LConn1
  L3/LConn1 -- Current Measurement2/RConn1 -- Controlled Current Source1/LConn1
  Diode1/RConn1 -- +VL/RConn1
  Current Measurement1/RConn1 -- Diode1/LConn1
  Current Measurement3/RConn1 -- Voltage Measurement/LConn1 -- Current Measurement1/LConn1 -- L1/LConn1
  Cotrolled Voltage Source1/RConn1 -- L2/RConn1
  Voltage Measurement1/LConn1 -- +VH/RConn1 -- Diode2/LConn1
  L3/RConn1 -- Controlled Current Source1/RConn1 -- Voltage Measurement/LConn2 -- -VL/RConn1 -- L1/RConn1 -- Cotrolled Voltage Source1/LConn1 -- Voltage Measurement1/LConn2 -- -VH/RConn1

== system power_FCHPS_MEA/Fuel Cell Power Module (FCPM)/Contactors1 ==
  Series RLC Branch1 : powerlib/Elements/Series RLC Branch  LConnTagsString=__new0  RConnTagsString=__new0  BranchType=R  Resistance=0.018  Inductance=1e-3  SetiL0=off  InitialCurrent=0  Capacitance=1e-6  Setx0=off  InitialVoltage=0  Measurements=None
  A : PMIOPort  Side=Left
  B : PMIOPort  Port=2  Side=Right
  connections:
  Series RLC Branch1/RConn1 -- B/RConn1
  A/RConn1 -- Series RLC Branch1/LConn1

== system power_FCHPS_MEA/Fuel Cell Power Module (FCPM)/FCPM Controller ==
  IFC : Inport
  Add : Sum
  Air blower delay2 : TransferFcn  Denominator=[0.33 1]
  Bus Selector1 : BusSelector  OutputSignals=Current
  Constant2 : Constant  Value=30
  Flow rate regulator Air : Subsystem
  Flow rate regulator H2 : Subsystem
  IFCmax : Outport  VectorParamsAs1DForOutWhenUnconnected=off
  AirFr : Outport  Port=2  VectorParamsAs1DForOutWhenUnconnected=off
  H2Fr : Outport  Port=3  VectorParamsAs1DForOutWhenUnconnected=off
  wires:
  Flow rate regulator Air/1(flow rate) -> Air blower delay2/1
  Constant2/1 -> Add/2
  Flow rate regulator H2/1(flow rate) -> H2Fr/1
  Add/1 -> IFCmax/1
  IFC/1 -> Bus Selector1/1
  Bus Selector1/1 -> Flow rate regulator H2/1(Iref), Flow rate regulator Air/1(Iref), Add/1  "<Current>"
  Air blower delay2/1 -> AirFr/1

== system power_FCHPS_MEA/3-phase AC load/Dynamic Impedance/Impedance Calculation ==
  S : Inport
  Constant7 : Constant  Value=(115*sqrt(2))^2
  Divide1 : Product  Inputs=/*
  conjugate : Math  Operator=conj  SignedPower=on  SaturateOnIntegerOverflow=on
  Z : Outport  VectorParamsAs1DForOutWhenUnconnected=off
  wires:
  Divide1/1 -> conjugate/1
  Constant7/1 -> Divide1/2
  S/1 -> Divide1/1
  conjugate/1 -> Z/1

== system power_FCHPS_MEA/DC//DC Boost Converter/DC//DC Boost Converter/Discrete PI Controller1 ==
  note: Discrete PID Controller
  note: Pierre Giroux, Gilbert Sybille
      | Power System Simulation Laboratory
      | IREQ, Hydro-Quebc
  Error : Inport  SampleTime=Ts
  Discrete-Time Integrator : DiscreteIntegrator  InitialCondition=Init  SampleTime=Ts  LimitOutput=on  UpperSaturationLimit=UpperLimit  LowerSaturationLimit=LowerLimit  ICPrevOutput=DiscIntNeverNeededParam  ICPrevScaledInput=DiscIntNeverNeededParam
  Kp4 : Gain  Gain=Kp  SaturateOnIntegerOverflow=on  SampleTime=Ts  OutDataTypeStr=Inherit: Same as input  ParamDataTypeStr=Inherit: Same as input
  Kp5 : Gain  Gain=Ki  SaturateOnIntegerOverflow=on  SampleTime=Ts  OutDataTypeStr=Inherit: Same as input  ParamDataTypeStr=Inherit: Same as input
  Saturation2 : Saturate  UpperLimit=UpperLimit  LowerLimit=LowerLimit  SampleTime=Ts
  Sum6 : Sum  InputSameDT=on  SaturateOnIntegerOverflow=on  SampleTime=Ts  OutDataTypeStr=Inherit: Same as first input
  Zero-Order Hold : ZeroOrderHold  SampleTime=Ts
  Out : Outport  SampleTime=Ts  InitialOutput=0  VectorParamsAs1DForOutWhenUnconnected=off
  wires:
  Zero-Order Hold/1 -> Sum6/1
  Saturation2/1 -> Out/1
  Discrete-Time Integrator/1 -> Sum6/2
  Kp4/1 -> Zero-Order Hold/1
  Kp5/1 -> Discrete-Time Integrator/1
  Sum6/1 -> Saturation2/1
  Error/1 -> Kp5/1, Kp4/1

== system power_FCHPS_MEA/DC//DC Boost Converter/DC//DC Boost Converter/Discrete PI Controller2 ==
  note: Pierre Giroux, Gilbert Sybille
      | Power System Simulation Laboratory
      | IREQ, Hydro-Quebc
  note: Discrete PID Controller
  Error : Inport  SampleTime=Ts
  Discrete-Time Integrator : DiscreteIntegrator  InitialCondition=Init  SampleTime=Ts  LimitOutput=on  UpperSaturationLimit=UpperLimit  LowerSaturationLimit=LowerLimit  ICPrevOutput=DiscIntNeverNeededParam  ICPrevScaledInput=DiscIntNeverNeededParam
  Kp4 : Gain  Gain=Kp  SaturateOnIntegerOverflow=on  SampleTime=Ts  OutDataTypeStr=Inherit: Same as input  ParamDataTypeStr=Inherit: Same as input
  Kp5 : Gain  Gain=Ki  SaturateOnIntegerOverflow=on  SampleTime=Ts  OutDataTypeStr=Inherit: Same as input  ParamDataTypeStr=Inherit: Same as input
  Saturation2 : Saturate  UpperLimit=UpperLimit  LowerLimit=LowerLimit  SampleTime=Ts
  Sum6 : Sum  InputSameDT=on  SaturateOnIntegerOverflow=on  SampleTime=Ts  OutDataTypeStr=Inherit: Same as first input
  Zero-Order Hold : ZeroOrderHold  SampleTime=Ts
  Out : Outport  SampleTime=Ts  InitialOutput=0  VectorParamsAs1DForOutWhenUnconnected=off
  wires:
  Error/1 -> Kp4/1, Kp5/1
  Sum6/1 -> Saturation2/1
  Kp5/1 -> Discrete-Time Integrator/1
  Kp4/1 -> Zero-Order Hold/1
  Discrete-Time Integrator/1 -> Sum6/2
  Saturation2/1 -> Out/1
  Zero-Order Hold/1 -> Sum6/1

== system power_FCHPS_MEA/DC//DC Boost Converter/DC//DC Buck Converter For DC bus precharge/Discrete PI Controller1 ==
  note: Discrete PID Controller
  note: Pierre Giroux, Gilbert Sybille
      | Power System Simulation Laboratory
      | IREQ, Hydro-Quebc
  Error : Inport  SampleTime=Ts
  Discrete-Time Integrator : DiscreteIntegrator  InitialCondition=Init  SampleTime=Ts  LimitOutput=on  UpperSaturationLimit=UpperLimit  LowerSaturationLimit=LowerLimit  ICPrevOutput=DiscIntNeverNeededParam  ICPrevScaledInput=DiscIntNeverNeededParam
  Kp4 : Gain  Gain=Kp  SaturateOnIntegerOverflow=on  SampleTime=Ts  OutDataTypeStr=Inherit: Same as input  ParamDataTypeStr=Inherit: Same as input
  Kp5 : Gain  Gain=Ki  SaturateOnIntegerOverflow=on  SampleTime=Ts  OutDataTypeStr=Inherit: Same as input  ParamDataTypeStr=Inherit: Same as input
  Saturation2 : Saturate  UpperLimit=UpperLimit  LowerLimit=LowerLimit  SampleTime=Ts
  Sum6 : Sum  InputSameDT=on  SaturateOnIntegerOverflow=on  SampleTime=Ts  OutDataTypeStr=Inherit: Same as first input
  Zero-Order Hold : ZeroOrderHold  SampleTime=Ts
  Out : Outport  SampleTime=Ts  InitialOutput=0  VectorParamsAs1DForOutWhenUnconnected=off
  wires:
  Zero-Order Hold/1 -> Sum6/1
  Saturation2/1 -> Out/1
  Discrete-Time Integrator/1 -> Sum6/2
  Kp4/1 -> Zero-Order Hold/1
  Kp5/1 -> Discrete-Time Integrator/1
  Sum6/1 -> Saturation2/1
  Error/1 -> Kp5/1, Kp4/1

== system power_FCHPS_MEA/DC//DC Boost Converter/DC//DC Buck Converter For DC bus precharge/Discrete PI Controller2 ==
  note: Pierre Giroux, Gilbert Sybille
      | Power System Simulation Laboratory
      | IREQ, Hydro-Quebc
  note: Discrete PID Controller
  Error : Inport  SampleTime=Ts
  Discrete-Time Integrator : DiscreteIntegrator  InitialCondition=Init  SampleTime=Ts  LimitOutput=on  UpperSaturationLimit=UpperLimit  LowerSaturationLimit=LowerLimit  ICPrevOutput=DiscIntNeverNeededParam  ICPrevScaledInput=DiscIntNeverNeededParam
  Kp4 : Gain  Gain=Kp  SaturateOnIntegerOverflow=on  SampleTime=Ts  OutDataTypeStr=Inherit: Same as input  ParamDataTypeStr=Inherit: Same as input
  Kp5 : Gain  Gain=Ki  SaturateOnIntegerOverflow=on  SampleTime=Ts  OutDataTypeStr=Inherit: Same as input  ParamDataTypeStr=Inherit: Same as input
  Saturation2 : Saturate  UpperLimit=UpperLimit  LowerLimit=LowerLimit  SampleTime=Ts
  Sum6 : Sum  InputSameDT=on  SaturateOnIntegerOverflow=on  SampleTime=Ts  OutDataTypeStr=Inherit: Same as first input
  Zero-Order Hold : ZeroOrderHold  SampleTime=Ts
  Out : Outport  SampleTime=Ts  InitialOutput=0  VectorParamsAs1DForOutWhenUnconnected=off
  wires:
  Error/1 -> Kp4/1, Kp5/1
  Sum6/1 -> Saturation2/1
  Kp5/1 -> Discrete-Time Integrator/1
  Kp4/1 -> Zero-Order Hold/1
  Discrete-Time Integrator/1 -> Sum6/2
  Saturation2/1 -> Out/1
  Zero-Order Hold/1 -> Sum6/1

== system power_FCHPS_MEA/Energy Management System/FC DC//DC converter references/filter ==
  I : Inport
  Add2 : Sum
  Add3 : Sum  Inputs=+-
  Gain1 : Gain  Gain=Ts
  Gain2 : Gain  Gain=1.2
  Gain3 : Gain  Gain=1/1.2
  Unit Delay : UnitDelay  SampleTime=Ts  HasFrameUpgradeWarning=on
  If : Outport  VectorParamsAs1DForOutWhenUnconnected=off
  wires:
  Add3/1 -> Gain1/1
  Unit Delay/1 -> Add3/2, Gain2/1
  Gain3/1 -> Unit Delay/1, If/1
  Add2/1 -> Gain3/1
  Gain2/1 -> Add2/2
  Gain1/1 -> Add2/1
  I/1 -> Add3/1
